simulink model "ControlFuzzy_Planta_pid_GA"  (R2021b)
settings: Solver=VariableStepAuto  StartTime=0.0  StopTime=1200  RelTol=1e-3
undefined symbols (not defined in the file or in its folder): sigbuilder_block
libraries: fuzblock x1, realtime_pacer_lib x1
settings Model: Creator=diego  LastModifiedBy=diego
settings SolverCC: AlgebraicLoopSolver=TrustRegion
settings DataIOCC: SaveOutput=off  SaveTime=off
settings DebuggingCC: SFMachineParentedDataDiag=warning

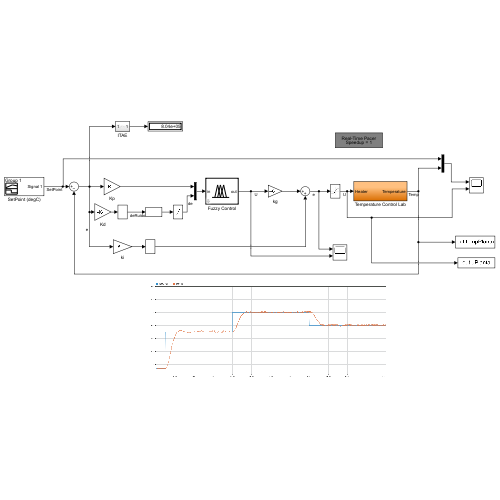
[thumbnail: Simulink's stored preview of the top-level diagram]
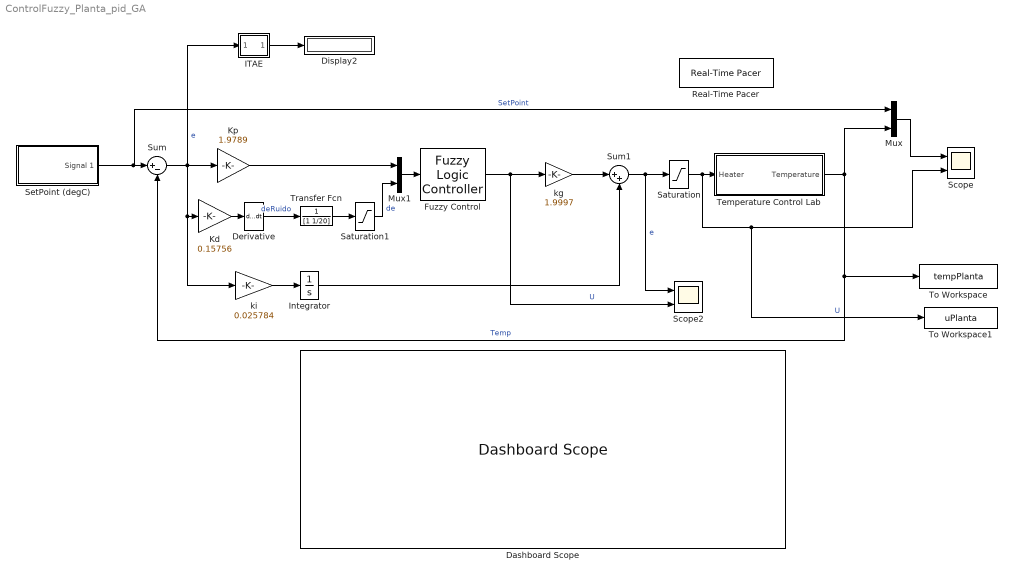
== system ControlFuzzy_Planta_pid_GA ==
  Dashboard Scope : DashboardScope  Ymin=23  Ymax=90  ScaleAtStop=off
  Derivative : Derivative
  Display2 : Display
  Fuzzy Control : fuzblock/Fuzzy Logic  Controller  FIS='C_Fuzzy_u100.fis'  OutputSampleNumber=101  DataType=double  FuzzifiedInputs=off  RuleFiringStrengths=off  RuleOutputs=off  AggregatedOutputs=off  SimulateUsing=Interpreted execution  OutOfRangeInputValueMessage=warning  NoRuleFiredMessage=warning  EmptyOutputFuzzySetMessage=warning
  ITAE : Subsystem
  Integrator : Integrator
  Kd : Gain  Gain=0.15756
  Kp : Gain  Gain=1.9789
  Mux : Mux  Inputs=2
  Mux1 : Mux  Inputs=2
  Real-Time Pacer : realtime_pacer_lib/Real-Time Pacer  simTimePerRealTime=1
  Saturation : Saturate  UpperLimit=100  LowerLimit=0
  Saturation1 : Saturate  UpperLimit=2  LowerLimit=-2
  Scope : Scope  NumInputPorts=2
  Scope2 : Scope  NumInputPorts=2
  SetPoint (degC) : Subsystem  Tag=STV Subsys  LoadFcn=sigbuilder_block('load');  StartFcn=sigbuilder_block('start');  StopFcn=sigbuilder_block('stop');  ClipboardFcn=sigbuilder_block('clipboard');  mask(Sigbuilder block){tuvar=[0:10]}
      mask help: Simulink:masks:SigbuilderBlock_MD
      mask init:
      | if ~strcmp(get_param(bdroot(gcbh),'SimulationStatus'),'stopped') tuvar = sigbuilder_block('maskInit'); end
      settings: CopyFcn=sigbuilder_block('copy');  DeleteFcn=sigbuilder_block('delete');  ModelCloseFcn=sigbuilder_block('modelClose');  PreSaveFcn=sigbuilder_block('preSave');  PauseFcn=sigbuilder_block('pause');  ContinueFcn=sigbuilder_block('continue');  NameChangeFcn=sigbuilder_block('namechange');  OpenFcn=sigbuilder_block('open',[53.4 0 1093.2 552.6 ]);  CloseFcn=sigbuilder_block('close');
      mask Display: plot(0, 0, 100, 100,[2, 2, 32, 32, 2], [68, 8, 8, 68, 68],[32, 2], [38, 38], [32, 19, 2],[53, 60, 44], [32, 17, 17, 2],[16, 16, 31, 31]);txt = getActiveGroup(gcbh);text(2, 100, txt,'verticalAlignment', 'top');
  Sum : Sum  Inputs=|+-
  Sum1 : Sum  Inputs=|++
  Temperature Control Lab : Subsystem
  To Workspace : ToWorkspace  VariableName=tempPlanta  SampleTime=1
      settings: Save2DSignal=2-D array (concatenate along first dimension)
  To Workspace1 : ToWorkspace  VariableName=uPlanta  SampleTime=1
      settings: Save2DSignal=2-D array (concatenate along first dimension)
  Transfer Fcn : TransferFcn  Denominator=[1 1/20]
  kg : Gain  Gain=1.9997
  ki : Gain  Gain=0.025784
  wires:
  Saturation/1 -> Temperature Control Lab/1(Heater), To Workspace1/1, Scope/2  "U"
  Temperature Control Lab/1(Temperature) -> Mux/2, To Workspace/1, Sum/2  "Temp"
  Mux/1 -> Scope/1
  Mux1/1 -> Fuzzy Control/1
  Saturation1/1 -> Mux1/2  "de"
  Sum/1 -> ITAE/1(In1), Kp/1, Kd/1, ki/1  "e"
  Derivative/1 -> Transfer Fcn/1  "deRuido"
  Transfer Fcn/1 -> Saturation1/1
  SetPoint (degC)/1(Signal 1) -> Mux/1, Sum/1  "SetPoint"
  Fuzzy Control/1 -> kg/1, Scope2/2  "U"
  ki/1 -> Integrator/1
  kg/1 -> Sum1/1
  Sum1/1 -> Scope2/1, Saturation/1  "e"
  Integrator/1 -> Sum1/2
  Kd/1 -> Derivative/1
  Kp/1 -> Mux1/1
  ITAE/1(Out1) -> Display2/1

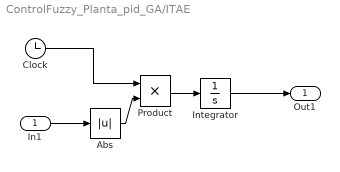
== system ControlFuzzy_Planta_pid_GA/ITAE ==
  In1 : Inport
  Abs : Abs
  Clock : Clock
  Integrator : Integrator
  Product : Product
  Out1 : Outport
  wires:
  Integrator/1 -> Out1/1
  Product/1 -> Integrator/1
  In1/1 -> Abs/1
  Clock/1 -> Product/1
  Abs/1 -> Product/2

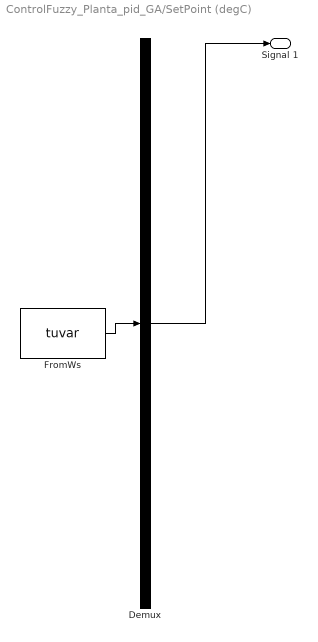
== system ControlFuzzy_Planta_pid_GA/SetPoint (degC) ==
  Demux : Demux  Tag=STV Demux  Outputs=1
      settings: DisplayOption=none
  FromWs : FromWorkspace  Tag=STV FromWs  VariableName=tuvar
      SigBuilderData=|
      | common.afterFinalStr = 'Extrapolate'
      | common.sampleTime = 0
      | dataSet.timeRange = [0 1200]
      | dataSet.name = 'Group 1'
      | sbobj.Groups.Name = 'Group 1'
      | sbobj.Groups.Signals.Name = 'Signal 1'
      | sbobj.Groups.Signals.XData = [0 50 50 400 400 800 800 1200]
      | sbobj.Groups.Signals.YData = [27 27 55 55 70.1 70.1 60 60]
      | sbobj.Groups.TimeRange = [0 1200]
  Signal 1 : Outport  Tag=STV Outport
  wires:
  Demux/1 -> Signal 1/1
  FromWs/1 -> Demux/1

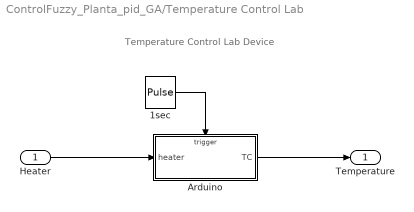
== system ControlFuzzy_Planta_pid_GA/Temperature Control Lab ==
  note: Temperature Control Lab Device
  Heater : Inport
  1sec : DiscretePulseGenerator  PulseType=Time based  Period=1  PulseWidth=50
  Arduino : Subsystem  TreatAsAtomicUnit=on
  Temperature : Outport  VectorParamsAs1DForOutWhenUnconnected=off
  wires:
  1sec/1 -> Arduino/Trigger
  Arduino/1(TC) -> Temperature/1
  Heater/1 -> Arduino/1(heater)

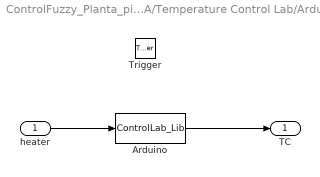
== system ControlFuzzy_Planta_pid_GA/Temperature Control Lab/Arduino ==
  heater : Inport  LatchByDelayingOutsideSignal=on
  Trigger : TriggerPort  VariantControl=Variant
  Arduino : MATLABFcn  MATLABFcn=ControlLab_Lib
  TC : Outport  InitialOutput=23  VectorParamsAs1DForOutWhenUnconnected=off
  wires:
  heater/1 -> Arduino/1
  Arduino/1 -> TC/1
